simulink library "casper_library"  (Simulink 6.5)
PostLoadFcn:
  | % Stub definitions for mask variables
  | delay_depth=16;
  | n_bits=8;
  | bin_pt=7;
values from neighbouring files (symbols this model uses):
  add_latency = get_var('add_latency', 'defaults', defaults, varargin{:})    [butterfly_direct_init.m]    (also in fft_direct_init.m; fft_init.m; fft_wideband_real_init.m; pfb_real_add_tree_init.m)
  BitWidthIn = get_var('BitWidthIn', 'defaults', defaults, varargin{:})    [pfb_real_add_tree_init.m]
  blockCountBits = ceil(log2(numBlocks))    [address_gen_vacc_v2_mask.m]
  blockRowBits = 0    [address_gen_vacc_v2_mask.m]
  CoeffBitWidth = get_var('CoeffBitWidth', 'defaults', defaults, varargin{:})    [pfb_coeff_gen_init.m]    (also in pfb_real_add_tree_init.m)
  mult_latency = get_var('mult_latency', 'defaults', defaults, varargin{:})    [butterfly_direct_init.m]    (also in fft_direct_init.m; fft_init.m; fft_wideband_real_init.m)
  n_inputs = get_var('n_inputs', 'defaults', defaults, varargin{:})    [fft_init.m]    (also in fft_unscrambler_init.m; fft_wideband_real_init.m; partial_delay_init.m = get_var('n_inputs', varargin{:}); pfb_coeff_gen_init.m)
  PFBSize = get_var('PFBSize', 'defaults', defaults, varargin{:})    [pfb_coeff_gen_init.m]
undefined symbols (not defined in the file or in its folder): acc_len, ant_bits, bit_growth, cmult_4bit_br, cmult_4bit_em, cmult_4bit_sl, n_ants, n_bits_out, num_ants
libraries: xbsIndex_r3 x1646, xbsIndex_r4 x226, casper_library x156, xbsReplacements_r4 x17, xps_library x10, fft_library x4
(part 2 of 14)

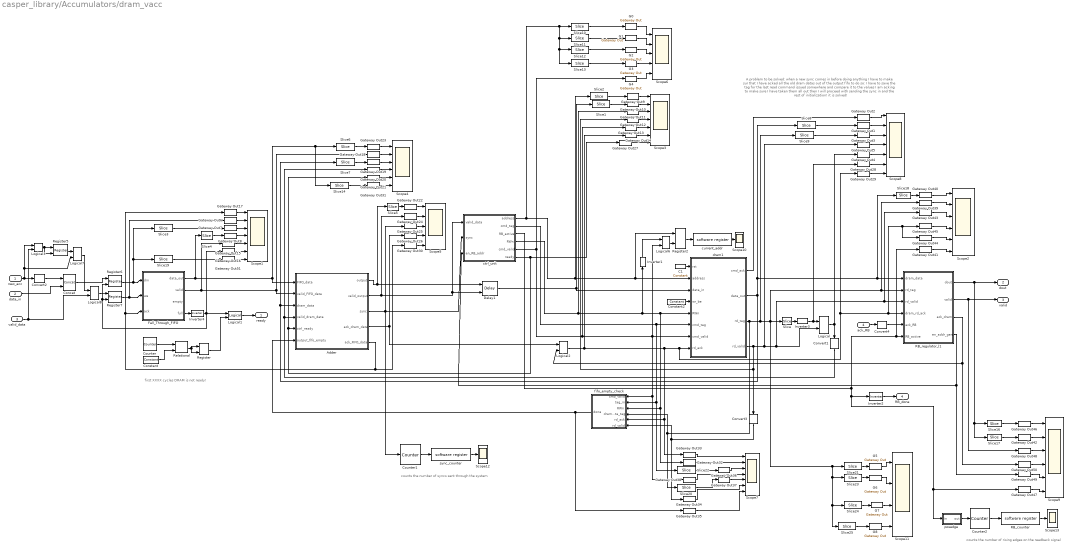
== system casper_library/Accumulators/dram_vacc ==
  note: A problem to be solved:
      | when a new sync comes in before doing anything I have to make sur
      | that I have acked all the old dram datas out of the output fifo
      | to do so: I have to save the tag for the last read command issued somewhere
      | and compare it to the values I am acking to make sure I have taken them all out
      | then I will proceed with sending the sync in and the rest of initialization!
      | it is solved!
  note: first XXXX cycles DRAM
      | is not ready!
  note: counts the number of syncs
      | sent through the system
  note: counts the number of rising edges on
      | the readback signal
  new_acc : Inport
  data_in : Inport  Port=2
  valid_data : Inport  Port=3
  ack_RB : Inport  Port=4
  Adder : Subsystem
  C1 : xbsIndex_r3/Constant  const=0  equ=P=C  arith_type=Boolean  n_bits=1  bin_pt=0  opselect=C  inp2=PCIN>>17  opr=+  inp1=P  carry=CIN  iostate=0  explicit_period=on  period=1  dbl_ovrd=off
  Concat : xbsIndex_r3/Concat  num_inputs=2  explicit_period=off  period=1  dbl_ovrd=off
  Constant : xbsIndex_r3/Constant  const=2^28-1  equ=P=C  arith_type=Unsigned  n_bits=28  bin_pt=0  opselect=C  inp2=PCIN>>17  opr=+  inp1=P  carry=CIN  iostate=0  explicit_period=on  period=1  dbl_ovrd=off
  Constant2 : xbsIndex_r3/Constant  const=2^18-1  equ=P=C  arith_type=Unsigned  n_bits=18  bin_pt=0  opselect=C  inp2=PCIN>>17  opr=+  inp1=P  carry=CIN  iostate=0  explicit_period=on  period=1  dbl_ovrd=off
  Convert1 : xbsIndex_r3/Convert  Orientation=down  arith_type=Boolean  n_bits=31  bin_pt=0  quantization=Truncate  overflow=Wrap  latency=0  explicit_period=off  period=1  dbl_ovrd=off  show_param=off  inserted_by_tool=off  pipeline=off
      settings: xl_area=[0, 0, 0, 0, 0, 0, 0]
  Convert2 : xbsIndex_r3/Convert  arith_type=Unsigned  n_bits=1  bin_pt=0  quantization=Truncate  overflow=Wrap  latency=0  explicit_period=off  period=1  dbl_ovrd=off  show_param=off  inserted_by_tool=off  pipeline=off
      settings: xl_area=[0, 0, 0, 0, 0, 0, 0]
  Convert3 : xbsIndex_r3/Convert  Orientation=down  arith_type=Boolean  n_bits=31  bin_pt=0  quantization=Truncate  overflow=Wrap  latency=0  explicit_period=off  period=1  dbl_ovrd=off  show_param=off  inserted_by_tool=off  pipeline=off
      settings: xl_area=[0, 0, 0, 0, 0, 0, 0]
  Convert4 : xbsIndex_r3/Convert  arith_type=Boolean  n_bits=31  bin_pt=0  quantization=Truncate  overflow=Wrap  latency=0  explicit_period=off  period=1  dbl_ovrd=off  show_param=off  inserted_by_tool=off  pipeline=off
      settings: xl_area=[0, 0, 0, 0, 0, 0, 0]
  Counter : xbsIndex_r3/Counter  cnt_type=Free Running  n_bits=28  bin_pt=0  arith_type=Unsigned  start_count=0  cnt_to=Inf  cnt_by_val=1  operation=Up  explicit_period=off  period=1  load_pin=off  rst=off  en=off  dbl_ovrd=off  show_param=off  use_rpm=on  gen_core=off
      settings: xl_area=[0, 0, 0, 0, 0, 0, 0]
  Counter1 : xbsIndex_r3/Counter  cnt_type=Free Running  n_bits=10  bin_pt=0  arith_type=Unsigned  start_count=0  cnt_to=Inf  cnt_by_val=1  operation=Up  explicit_period=off  period=1  load_pin=off  rst=off  en=on  dbl_ovrd=off  show_param=off  use_rpm=on  gen_core=off
      settings: xl_area=[0, 0, 0, 0, 0, 0, 0]
  Counter2 : xbsIndex_r3/Counter  cnt_type=Free Running  n_bits=10  bin_pt=0  arith_type=Unsigned  start_count=0  cnt_to=Inf  cnt_by_val=1  operation=Up  explicit_period=off  period=1  load_pin=off  rst=off  en=on  dbl_ovrd=off  show_param=off  use_rpm=on  gen_core=off
      settings: xl_area=[0, 0, 0, 0, 0, 0, 0]
  Delay1 : xbsIndex_r3/Delay  latency=1  reg_retiming=off  explicit_period=on  period=1  en=on  accept_only_valid=off  init_zero=on  dbl_ovrd=off  show_param=off
      settings: xl_area=[0, 0, 0, 0, 0, 0, 0]
  Fall_Through_FIFO : Subsystem
  G{0..8} (9 alike) : xbsIndex_r3/Gateway Out  output_type=Double  nbits=8  bin_pt=6  arith_type=Boolean  quantization=Truncate  overflow=Wrap  hdl_port=off  timing_constraint=None  locs_specified=off  LOCs={}  needs_fixed_name=off  show_param=off
      settings: xl_area=[0, 0, 0, 0, 0, 0, 0]
  Gateway Out{1..51} (51 alike) : xbsIndex_r3/Gateway Out  output_type=Double  nbits=8  bin_pt=6  arith_type=Boolean  quantization=Truncate  overflow=Wrap  hdl_port=off  timing_constraint=None  locs_specified=off  LOCs={}  needs_fixed_name=off  show_param=off
      settings: xl_area=[0, 0, 0, 0, 0, 0, 0]
  Inverter1 : xbsIndex_r3/Inverter  Orientation=up  latency=0  explicit_period=off  period=1  en=off  dbl_ovrd=off  show_param=off
      settings: xl_area=[0, 0, 0, 0, 0, 0, 0]
  Inverter2 : xbsIndex_r3/Inverter  latency=0  explicit_period=off  period=1  en=off  dbl_ovrd=off  show_param=off
      settings: xl_area=[0, 0, 0, 0, 0, 0, 0]
  Inverter3 : xbsIndex_r3/Inverter  latency=0  explicit_period=off  period=1  en=off  dbl_ovrd=off  show_param=off
      settings: xl_area=[0, 0, 0, 0, 0, 0, 0]
  Inverter4 : xbsIndex_r3/Inverter  latency=0  explicit_period=off  period=1  en=off  dbl_ovrd=off  show_param=off
      settings: xl_area=[0, 0, 0, 0, 0, 0, 0]
  Logical{,1,3,6,8} (5 alike) : xbsIndex_r3/Logical  logical_function=AND  inputs=2  precision=Full  arith_type=Unsigned  n_bits=8  bin_pt=2  align_bp=on  latency=0  explicit_period=off  period=1  en=off  dbl_ovrd=off  show_param=off
      settings: xl_area=[0, 0, 0, 0, 0, 0, 0]
  Logical2 : xbsIndex_r3/Logical  logical_function=OR  inputs=2  precision=Full  arith_type=Unsigned  n_bits=8  bin_pt=2  align_bp=on  latency=0  explicit_period=off  period=1  en=off  dbl_ovrd=off  show_param=off
      settings: xl_area=[0, 0, 0, 0, 0, 0, 0]
  Logical7 : xbsIndex_r3/Logical  logical_function=OR  inputs=2  precision=Full  arith_type=Unsigned  n_bits=8  bin_pt=2  align_bp=on  latency=0  explicit_period=off  period=1  en=off  dbl_ovrd=off  show_param=off
      settings: xl_area=[0, 0, 0, 0, 0, 0, 0]
  RB_counter : xps_library/software register  Tag=xps:sw_reg  io_dir=To Processor  arith_type=Unsigned  bitwidth=32  bin_pt=0  sample_period=1  gw_name=casper_library_Accumulators_dram_vacc_RB_counter_user_data_in
  RB_regulator_l1 : Subsystem
  Register{,2,5..7} (5 alike) : xbsIndex_r3/Register  init=0  reg_only_valid=off  explicit_period=off  period=1  rst=off  en=on  out_en=off  dbl_ovrd=off  show_param=off
      settings: xl_area=[0, 0, 0, 0, 0, 0, 0]
  Relational : xbsIndex_r3/Relational  mode=a=b  latency=1  explicit_period=off  period=1  en=off  dbl_ovrd=off  show_param=off
      settings: xl_area=[0, 0, 0, 0, 0, 0, 0]
  Scope{1,3,7..8} (4 alike) : Scope  NumInputPorts=7
      Scope1 settings: TimeRange=400000  YMin=0~0~0~0~0~0~0  YMax=1~1~400~400~1~2~1  SaveName=ScopeData7
      Scope3 settings: YMin=0~0~0~0~0~0~0  YMax=150~2500~1~1~1~1~1  SaveName=ScopeData6
      Scope7 settings: YMin=0~0~0~0~0~0.95~0  YMax=1~1100~7500~1~1~1.05~1  SaveName=ScopeData17
      Scope8 settings: YMin=0~0~2.68438e+008~0~0~0~0  YMax=1~11000~2.68439e+008~1~1~1~1  SaveName=ScopeData19
  Scope10 : Scope
      settings: YMin=0  YMax=100  SaveName=ScopeData27
  Scope11 : Scope  NumInputPorts=4
      settings: YMin=0~0~0~0  YMax=200~4000~1~1  SaveName=ScopeData28
  Scope12 : Scope
      settings: YMin=0  YMax=100  SaveName=ScopeData32
  Scope13 : Scope
      settings: YMin=0  YMax=100  SaveName=ScopeData33
  Scope2 : Scope  NumInputPorts=6
      settings: YMin=-1~0.95~-1~-1~0.95~-1  YMax=1~1.05~1~1~1.05~1  SaveName=ScopeData22
  Scope4 : Scope  NumInputPorts=6
      settings: YMin=0.95~0.95~-1~-1~0.95~-1  YMax=1.05~1.05~1~1~1.05~1  SaveName=ScopeData8
  Scope5 : Scope  NumInputPorts=5
      settings: YMin=0~0~-1~0~0  YMax=250~1~1~1~1  SaveName=ScopeData9
  Scope6 : Scope  NumInputPorts=5
      settings: YMin=0~0~0~0~0  YMax=200~4000~1~1~1  SaveName=ScopeData14
  Scope9 : Scope  NumInputPorts=6
      settings: YMin=1.9~1.9~-1~0~-1~0.95  YMax=2.1~2.1~1~1~1~1.05  SaveName=ScopeData23
  Slice : xbsIndex_r3/Slice  mode=Upper Bit Location + Width  nbits=1  bit1=0  base1=MSB of Input  bit0=0  base0=LSB of Input  boolean_output=off  explicit_period=off  period=1  dbl_ovrd=off
  Slice{1,3..8,16..18} (10 alike) : xbsIndex_r3/Slice  mode=Lower Bit Location + Width  nbits=32  bit1=0  base1=MSB of Input  bit0=0  base0=LSB of Input  boolean_output=off  explicit_period=off  period=1  dbl_ovrd=off
  Slice{2,10,20..22} (5 alike) : xbsIndex_r3/Slice  mode=Lower Bit Location + Width  nbits=8  bit1=0  base1=MSB of Input  bit0=5  base0=LSB of Input  boolean_output=off  explicit_period=off  period=1  dbl_ovrd=off
  Slice11 : xbsIndex_r3/Slice  mode=Lower Bit Location + Width  nbits=14  bit1=0  base1=MSB of Input  bit0=14  base0=LSB of Input  boolean_output=off  explicit_period=off  period=1  dbl_ovrd=off
  Slice12 : xbsIndex_r3/Slice  mode=Lower Bit Location + Width  nbits=1  bit1=0  base1=MSB of Input  bit0=13  base0=LSB of Input  boolean_output=off  explicit_period=off  period=1  dbl_ovrd=off
  Slice13 : xbsIndex_r3/Slice  mode=Lower Bit Location + Width  nbits=2  bit1=0  base1=MSB of Input  bit0=28  base0=LSB of Input  boolean_output=off  explicit_period=off  period=1  dbl_ovrd=off
  Slice14 : xbsIndex_r3/Slice  mode=Upper Bit Location + Width  nbits=1  bit1=0  base1=MSB of Input  bit0=0  base0=LSB of Input  boolean_output=off  explicit_period=off  period=1  dbl_ovrd=off
  Slice19 : xbsIndex_r3/Slice  mode=Upper Bit Location + Width  nbits=1  bit1=0  base1=MSB of Input  bit0=0  base0=LSB of Input  boolean_output=off  explicit_period=off  period=1  dbl_ovrd=off
  Slice23 : xbsIndex_r3/Slice  mode=Lower Bit Location + Width  nbits=14  bit1=0  base1=MSB of Input  bit0=14  base0=LSB of Input  boolean_output=off  explicit_period=off  period=1  dbl_ovrd=off
  Slice24 : xbsIndex_r3/Slice  mode=Lower Bit Location + Width  nbits=1  bit1=0  base1=MSB of Input  bit0=13  base0=LSB of Input  boolean_output=off  explicit_period=off  period=1  dbl_ovrd=off
  Slice25 : xbsIndex_r3/Slice  mode=Lower Bit Location + Width  nbits=2  bit1=0  base1=MSB of Input  bit0=28  base0=LSB of Input  boolean_output=off  explicit_period=off  period=1  dbl_ovrd=off
  Slice9 : xbsIndex_r3/Slice  mode=Lower Bit Location + Width  nbits=31  bit1=0  base1=MSB of Input  bit0=0  base0=LSB of Input  boolean_output=off  explicit_period=off  period=1  dbl_ovrd=off
  ctrl_unit : Subsystem  mask{burst_length=valid_length, acc_length=acc_length}
      mask prompts: burst_length "Burst Length?"; acc_length "Accumulation length?"
  current_addr : xps_library/software register  Tag=xps:sw_reg  io_dir=To Processor  arith_type=Unsigned  bitwidth=32  bin_pt=0  sample_period=1  gw_name=casper_library_Accumulators_dram_vacc_current_addr_user_data_in
  dram1 : Subsystem  Tag=xps:dram  AncestorBlock=xps_library/dram  mask(dram){dimm=1, arith_type=Unsigned, bin_pt=0, ip_clock=200, sample_period=1, use_sim=on, bank_mgt=on, wide_data=off, half_burst=off, shared=on}
      mask prompts: arith_type "Data Type"; bin_pt "Data binary point"; ip_clock "Datapath clock rate (MHz)"; sample_period "Sample period"; use_sim "Simulate DRAM using ModelSim"; bank_mgt "Enable bank management"; wide_data "Use wide data bus (288 bits)"; half_burst "Use half-burst"; shared "Share with PowerPC"
      mask help:
      | Interface to 1GB DDR2 DIMMs on BEE2.
      |
      | To simulate using ModelSim, place a ModelSim block named 'ModelSim' (case-sensitive) in the top level of the design.
      mask init:
      | dram_mask;
      mask StyleString: popup(1|2|3|4),popup(Boolean|Unsigned|Signed  (2's comp)),edit,edit,edit,checkbox,checkbox,checkbox,checkbox,checkbox
      mask CallbackString:
      | |||||||myname=gcb;
      | if strcmp(get_param(myname, 'wide_data'), 'off')
      |     set_param(myname, 'MaskEnables', {'on','on','on','on','on','on','on','on','on','on'});
      | else
      |     set_param(myname, 'half_burst', 'off');
      |     set_param(myname, 'MaskEnables', {'on','on','on','on','on','on','on','on','off','on'});
      | end||
  fifo_empty_check : Subsystem  Orientation=left
  posedge : Subsystem
  sync_counter : xps_library/software register  Tag=xps:sw_reg  io_dir=To Processor  arith_type=Unsigned  bitwidth=32  bin_pt=0  sample_period=1  gw_name=casper_library_Accumulators_dram_vacc_sync_counter_user_data_in
  ready : Outport
  dout : Outport  Port=2
  valid : Outport  Port=3
  RB_done : Outport  Port=4
  wires:
  Logical8/1 -> Register7/1
  Concat/1 -> Register6/1
  Logical3/1 -> Register5/2, Register5/1
  Logical7/1 -> Logical8/1
  Register5/1 -> Logical7/1
  Convert2/1 -> Concat/1
  valid_data/1 -> Logical8/2, Logical3/2
  data_in/1 -> Concat/2
  new_acc/1 -> Logical3/1, Logical7/2, Convert2/1
  Adder/4(ack_dram_data) -> Gateway Out26/1, Logical2/1
  Fall_Through_FIFO/1(data_out) -> Adder/1(FIFO_data), Slice6/1, Slice14/1, Slice4/1
  Fall_Through_FIFO/2(valid) -> Gateway Out15/1, Gateway Out18/1, Adder/2(valid_FIFO_data)
  ctrl_unit/1(address) -> Slice10/1, Slice11/1, Slice13/1, Slice12/1, Slice2/1, dram1/2(address), Register2/1
  ctrl_unit/4(RWn) -> Gateway Out11/1, dram1/5(RWn), fifo_empty_check/3(RWn), Gateway Out32/1, Inverter1/1
  C1/1 -> dram1/1(rst)
  Constant2/1 -> dram1/4(wr_be)
  Adder/1(output) -> Slice5/1, Delay1/1
  dram1/2(data_out) -> Slice7/1, Adder/3(dram_data), Slice8/1, Slice18/1, RB_regulator_l1/1(dram_data)
  dram1/3(rd_tag) -> Slice9/1, Slice/1, Slice21/1, Slice23/1, Slice25/1, Slice24/1, Gateway Out39/1, RB_regulator_l1/2(rd_tag), fifo_empty_check/4(dram_data_tag), Slice20/1
  Slice/1 -> Inverter3/1
  dram1/4(rd_valid) -> Gateway Out5/1, Logical/2, Gateway Out43/1, RB_regulator_l1/3(rd_valid), Gateway Out12/1, Convert3/1
  Logical/1 -> Gateway Out4/1, Convert1/1
  ctrl_unit/6(ready) -> Gateway Out21/1, Adder/5(ctrl_ready), Gateway Out27/1
  Adder/2(valid_output) -> ctrl_unit/1(valid_data), Delay1/2, Gateway Out24/1
  Adder/3(sync) -> Gateway Out25/1, Counter1/1, ctrl_unit/2(sync)
  dram1/1(cmd_ack) -> Gateway Out2/1
  ctrl_unit/2(cmd_tag) -> dram1/6(cmd_tag), fifo_empty_check/2(tag_in), Slice22/1
  Fall_Through_FIFO/4(full) -> Inverter4/1
  Register6/1 -> Fall_Through_FIFO/1(din), Slice3/1, Slice19/1
  Gateway Out9/1 -> Scope3/1
  Gateway Out10/1 -> Scope3/2
  Gateway Out11/1 -> Scope3/3
  Gateway Out12/1 -> Scope3/4
  Gateway Out13/1 -> Scope3/5
  Gateway Out14/1 -> Scope3/6
  Slice1/1 -> Gateway Out10/1
  Slice2/1 -> Gateway Out9/1
  Gateway Out17/1 -> Scope1/1
  Gateway Out6/1 -> Scope1/2
  Gateway Out7/1 -> Scope1/3
  Gateway Out8/1 -> Scope1/4
  Gateway Out15/1 -> Scope1/5
  Gateway Out16/1 -> Scope1/6
  Gateway Out23/1 -> Scope4/1
  Gateway Out18/1 -> Scope4/2
  Gateway Out19/1 -> Scope4/3
  Gateway Out20/1 -> Scope4/4
  Gateway Out21/1 -> Scope4/5
  Gateway Out22/1 -> Scope5/1
  Gateway Out24/1 -> Scope5/2
  Gateway Out25/1 -> Scope5/3
  Gateway Out26/1 -> Scope5/4
  Slice3/1 -> Gateway Out7/1
  Slice4/1 -> Gateway Out8/1
  Convert1/1 -> Gateway Out20/1, Adder/4(valid_dram_data)
  Slice5/1 -> Gateway Out22/1
  Slice6/1 -> Gateway Out23/1
  Slice7/1 -> Gateway Out19/1
  Gateway Out27/1 -> Scope3/7
  Slice8/1 -> Gateway Out1/1
  Slice9/1 -> Gateway Out3/1
  Adder/5(ack_FIFO_data) -> Fall_Through_FIFO/3(ack), Gateway Out17/1, Gateway Out30/1
  Gateway Out30/1 -> Scope5/5
  Slice10/1 -> G0/1
  Slice11/1 -> G1/1
  Slice12/1 -> G2/1
  Slice13/1 -> G3/1
  G0/1 -> Scope6/1
  G1/1 -> Scope6/2
  G2/1 -> Scope6/3
  G3/1 -> Scope6/4
  G4/1 -> Scope6/5
  Gateway Out31/1 -> Scope4/6
  Slice14/1 -> Gateway Out31/1
  Delay1/1 -> dram1/3(data_in), Slice1/1
  fifo_empty_check/1(done) -> Adder/6(output_fifo_empty), Gateway Out35/1
  Gateway Out33/1 -> Scope7/1
  Gateway Out32/1 -> Scope7/2
  Gateway Out36/1 -> Scope7/3
  Gateway Out37/1 -> Scope7/5
  Gateway Out38/1 -> Scope7/4
  Gateway Out34/1 -> Scope7/6
  Gateway Out35/1 -> Scope7/7
  Gateway Out2/1 -> Scope8/1
  Gateway Out1/1 -> Scope8/2
  Gateway Out3/1 -> Scope8/3
  Gateway Out5/1 -> Scope8/4
  Gateway Out4/1 -> Scope8/5
  Gateway Out28/1 -> Scope8/6
  Gateway Out29/1 -> Scope8/7
  RB_regulator_l1/1(dout) -> dout/1, Slice16/1, Slice17/1
  RB_regulator_l1/2(valid) -> Gateway Out48/1, valid/1
  RB_regulator_l1/3(ack_dram) -> Gateway Out50/1, Logical2/2
  RB_regulator_l1/4(en_addr_gen) -> ctrl_unit/3(en_RB_addr), Gateway Out49/1
  ctrl_unit/3(RB_active) -> Gateway Out41/1, RB_regulator_l1/6(RB_active), Gateway Out47/1, posedge/1(in), Inverter2/1
  Logical2/1 -> fifo_empty_check/5(rd_ack), Gateway Out33/1, dram1/8(rd_ack), Gateway Out29/1, RB_regulator_l1/4(dram_rd_ack), Gateway Out45/1, Gateway Out44/1, Gateway Out14/1
  Gateway Out40/1 -> Scope2/1
  Gateway Out39/1 -> Scope2/2
  Gateway Out43/1 -> Scope2/3
  Gateway Out45/1 -> Scope2/4
  Gateway Out44/1 -> Scope2/5
  Gateway Out41/1 -> Scope2/6
  Gateway Out46/1 -> Scope9/1
  Gateway Out42/1 -> Scope9/2
  Gateway Out48/1 -> Scope9/3
  Gateway Out50/1 -> Scope9/4
  Gateway Out49/1 -> Scope9/5
  Convert3/1 -> fifo_empty_check/6(rd_valid), Gateway Out34/1
  Slice16/1 -> Gateway Out46/1
  Slice17/1 -> Gateway Out42/1
  Slice18/1 -> Gateway Out40/1
  Gateway Out47/1 -> Scope9/6
  Logical1/1 -> ready/1
  Counter/1 -> Relational/1
  Constant/1 -> Relational/2
  Relational/1 -> Register/1, Register/2
  Register/1 -> Logical1/2
  Register7/1 -> Fall_Through_FIFO/2(we), Gateway Out6/1
  Gateway Out51/1 -> Scope1/7
  Slice19/1 -> Gateway Out51/1
  Register2/1 -> current_addr/1
  Logical6/1 -> Register2/2
  Inverter1/1 -> Logical6/1
  current_addr/1 -> Scope10/1
  Slice22/1 -> Gateway Out36/1
  Slice20/1 -> Gateway Out37/1
  Slice21/1 -> G5/1
  Slice23/1 -> G6/1
  Slice24/1 -> G7/1
  Slice25/1 -> G8/1
  G5/1 -> Scope11/1
  G6/1 -> Scope11/2
  G7/1 -> Scope11/3
  G8/1 -> Scope11/4
  Inverter4/1 -> Register6/2, Register7/2, Gateway Out16/1, Logical1/1
  Counter1/1 -> sync_counter/1
  sync_counter/1 -> Scope12/1
  Counter2/1 -> RB_counter/1
  RB_counter/1 -> Scope13/1
  posedge/1(out) -> Counter2/1
  Inverter2/1 -> RB_done/1
  ctrl_unit/5(cmd_valid) -> Gateway Out13/1, dram1/7(cmd_valid), fifo_empty_check/1(cmd_valid), Gateway Out38/1, Logical6/2, G4/1
  ack_RB/1 -> Convert4/1
  Inverter3/1 -> Logical/1, Gateway Out28/1
  Convert4/1 -> RB_regulator_l1/5(ack_RB)

== system casper_library/Correlator/baseline_tap ==
  a_del : Inport
  a_ndel : Inport  Port=2
  a_end : Inport  Port=3
  acc_in : Inport  Port=4
  valid_in : Inport  Port=5
  rst : Inport  Port=6
  sync1 : Inport  Port=7
  Constant : xbsIndex_r3/Constant  const=ant_sep * acc_len  equ=P=C  arith_type=Unsigned  n_bits=ant_bits + bit_growth  bin_pt=0  opselect=C  inp2=PCIN>>17  opr=+  inp1=P  carry=CIN  iostate=0  explicit_period=off  period=1  dbl_ovrd=off
  Convert : xbsIndex_r3/Convert  arith_type=Unsigned  n_bits=1  bin_pt=0  quantization=Truncate  overflow=Wrap  latency=0  explicit_period=off  period=1  dbl_ovrd=off  show_param=off  inserted_by_tool=off  pipeline=off
      settings: xl_area=[0, 0, 0, 0, 0, 0, 0]
  Counter : xbsIndex_r3/Counter  cnt_type=Count Limited  n_bits=ant_bits + bit_growth  bin_pt=0  arith_type=Unsigned  start_count=0  cnt_to=n_ants * acc_len - 1  cnt_by_val=1  operation=Up  explicit_period=off  period=1  load_pin=off  rst=on  en=off  dbl_ovrd=off  show_param=off  use_rpm=on  gen_core=off
      settings: xl_area=[0, 0, 0, 0, 0, 0, 0]
  Delay1 : xbsIndex_r3/Delay  latency=1  reg_retiming=off  explicit_period=off  period=1  en=off  accept_only_valid=off  init_zero=on  dbl_ovrd=off  show_param=off
      settings: xl_area=[0, 0, 0, 0, 0, 0, 0]
  Delay3 : xbsIndex_r3/Delay  latency=1  reg_retiming=off  explicit_period=off  period=1  en=off  accept_only_valid=off  init_zero=on  dbl_ovrd=off  show_param=off
      settings: xl_area=[0, 0, 0, 0, 0, 0, 0]
  Delay7 : xbsIndex_r3/Delay  latency=1  reg_retiming=off  explicit_period=on  period=1  en=off  accept_only_valid=off  init_zero=on  dbl_ovrd=off  show_param=off
      settings: xl_area=[0, 0, 0, 0, 0, 0, 0]
  Delay8 : xbsIndex_r3/Delay  latency=1  reg_retiming=off  explicit_period=on  period=1  en=off  accept_only_valid=off  init_zero=on  dbl_ovrd=off  show_param=off
      settings: xl_area=[0, 0, 0, 0, 0, 0, 0]
  Mux : xbsIndex_r3/Mux  inputs=2  precision=Full  arith_type="Signed  (2's comp)"  n_bits=8  bin_pt=2  quantization=Truncate  overflow=Wrap  latency=1  explicit_period=off  period=1  en=off  dbl_ovrd=off  show_param=off  mux_type=off  use_rpm=off  gen_core=off
      settings: xl_area=[0, 0, 0, 0, 0, 0, 0]
  Relational : xbsIndex_r3/Relational  mode=a<b  latency=0  explicit_period=off  period=1  en=off  dbl_ovrd=off  show_param=off
      settings: xl_area=[0, 0, 0, 0, 0, 0, 0]
  delay : Subsystem  BlockChoice=delay_bram
      link override delay_bram: DelayLen=acc_len  bram_latency=bram_latency
      link override delay_slr: DelayLen=acc_len
      settings: AttributesFormatString=%<BlockChoice>  TemplateBlock=casper_library/Delays/delay  MemberBlocks=delay_bram,delay_slr
  dual_pol_cmac : Subsystem
  a_del_out : Outport
  a_ndel_out : Outport  Port=2
  a_end_out : Outport  Port=3
  acc_out : Outport  Port=4
  valid_out : Outport  Port=5
  rst_out : Outport  Port=6
  sync_out : Outport  Port=7
  wires:
  sync1/1 -> sync_out/1
  Delay1/1 -> rst_out/1, dual_pol_cmac/4(sync)
  Delay8/1 -> a_end_out/1
  Delay7/1 -> a_ndel_out/1
  Delay3/1 -> a_del_out/1, dual_pol_cmac/1(a1)
  a_end/1 -> Delay8/1, Mux/3
  a_ndel/1 -> Delay7/1, Mux/2
  valid_in/1 -> dual_pol_cmac/5(valid_in)
  dual_pol_cmac/2(valid_out) -> valid_out/1
  acc_in/1 -> dual_pol_cmac/3(acc_in)
  dual_pol_cmac/1(acc_out) -> acc_out/1
  a_del/1 -> delay/1(In1)
  rst/1 -> Counter/1, Delay1/1
  Convert/1 -> Mux/1
  Relational/1 -> Convert/1
  Constant/1 -> Relational/2
  Counter/1 -> Relational/1
  Mux/1 -> dual_pol_cmac/2(a2)
  delay/1(Out1) -> Delay3/1

== system casper_library/Correlator/x_engine ==
  ant : Inport
  sync_in : Inport  Port=2
  Constant : xbsIndex_r3/Constant  const=0  equ=P=C  arith_type=Unsigned  n_bits=8 * n_bits_out  bin_pt=0  opselect=C  inp2=PCIN>>17  opr=+  inp1=P  carry=CIN  iostate=0  explicit_period=on  period=1  dbl_ovrd=off
  Constant1 : xbsIndex_r3/Constant  const=0  equ=P=C  arith_type=Boolean  n_bits=1  bin_pt=0  opselect=C  inp2=PCIN>>17  opr=+  inp1=P  carry=CIN  iostate=0  explicit_period=on  period=1  dbl_ovrd=off
  Term1 : Terminator
  Term2 : Terminator
  Term3 : Terminator
  auto_tap : Subsystem  mask(auto_tap){use_ded_mult=1}
      mask prompts: use_ded_mult "Use Dedicated Multipliers"
      mask init:
      | auto_tap_init(gcb, ...
      |     'use_ded_mult', use_ded_mult);
      settings: AttributesFormatString=mult=1
  baseline_tap1 : casper_library/Correlator/baseline_tap  ant_sep=1  use_ded_mult=1  use_bram_delay=1
      settings: AttributesFormatString=ant_sep=1, mult=1, bram=1
  baseline_tap2 : casper_library/Correlator/baseline_tap  ant_sep=2  use_ded_mult=1  use_bram_delay=1
      settings: AttributesFormatString=ant_sep=2, mult=1, bram=1
  acc : Outport
  valid : Outport  Port=2
  sync_out : Outport  Port=3
  wires:
  ant/1 -> auto_tap/1(a_del), auto_tap/2(a_ndel)
  Constant/1 -> auto_tap/4(acc_in)
  Constant1/1 -> auto_tap/5(valid_in)
  sync_in/1 -> auto_tap/6(sync_in)
  auto_tap/1(a_del_out) -> baseline_tap1/1
  auto_tap/2(a_ndel_out) -> baseline_tap1/2
  auto_tap/3(a_end_out) -> baseline_tap1/3
  auto_tap/4(acc_out) -> baseline_tap1/4
  auto_tap/5(valid_out) -> baseline_tap1/5
  auto_tap/6(rst_out) -> baseline_tap1/6
  auto_tap/7(sync_out) -> baseline_tap1/7
  baseline_tap1/1 -> baseline_tap2/1
  baseline_tap1/2 -> baseline_tap2/2
  baseline_tap1/3 -> baseline_tap2/3
  baseline_tap1/4 -> baseline_tap2/4
  baseline_tap1/5 -> baseline_tap2/5
  baseline_tap1/6 -> baseline_tap2/6
  baseline_tap1/7 -> baseline_tap2/7
  baseline_tap2/1 -> auto_tap/3(a_loop)
  baseline_tap2/2 -> Term1/1
  baseline_tap2/3 -> Term2/1
  baseline_tap2/4 -> acc/1
  baseline_tap2/5 -> valid/1
  baseline_tap2/6 -> Term3/1
  baseline_tap2/7 -> sync_out/1

== system casper_library/Correlator/x_engine_reorder ==
  acc : Inport
  valid : Inport  Port=2
  window_valid : Inport  Port=3
  sync : Inport  Port=4
  Constant4 : xbsIndex_r3/Constant  const=0  equ=P=C  arith_type=Boolean  n_bits=elements_bits + 1  bin_pt=0  opselect=C  inp2=PCIN>>17  opr=+  inp1=P  carry=CIN  iostate=0  explicit_period=on  period=1  dbl_ovrd=off
  Counter1 : xbsIndex_r3/Counter  cnt_type=Count Limited  n_bits=elements_bits + 1  bin_pt=0  arith_type=Unsigned  start_count=0  cnt_to=2 * num_elements - 1  cnt_by_val=1  operation=Up  explicit_period=off  period=1  load_pin=off  rst=on  en=on  dbl_ovrd=off  show_param=off  use_rpm=on  gen_core=off
      settings: xl_area=[0, 0, 0, 0, 0, 0, 0]
  Delay{1..3,6,8} (5 alike) : xbsIndex_r3/Delay  latency=1  reg_retiming=off  explicit_period=off  period=1  en=off  accept_only_valid=off  init_zero=on  dbl_ovrd=off  show_param=off
      settings: xl_area=[0, 0, 0, 0, 0, 0, 0]
  Dual Port RAM : xbsIndex_r3/Dual Port RAM  depth=num_elements * 2  initVector=0  write_mode_A=Read After Write  write_mode_B=No Read On Write  latency=1  mem_collision=off  init_zero=on  explicit_period=off  period=1  dbl_ovrd=off  rst_a=off  init_a=0  rst_b=off  init_b=0  show_param=off  distributed_mem=off  use_rpm=off  gen_core=off
      settings: xl_area=[0, 0, 0, 0, 0, 0, 0]
  Logical{,1,4,7} (4 alike) : xbsIndex_r3/Logical  logical_function=OR  inputs=2  precision=Full  arith_type=Unsigned  n_bits=8  bin_pt=2  align_bp=on  latency=0  explicit_period=off  period=1  en=off  dbl_ovrd=off  show_param=off
      settings: xl_area=[0, 0, 0, 0, 0, 0, 0]
  Mux : xbsIndex_r3/Mux  inputs=2  precision=Full  arith_type="Signed  (2's comp)"  n_bits=8  bin_pt=2  quantization=Truncate  overflow=Wrap  latency=0  explicit_period=off  period=1  en=off  dbl_ovrd=off  show_param=off  mux_type=off  use_rpm=off  gen_core=off
      settings: xl_area=[0, 0, 0, 0, 0, 0, 0]
  Terminator : Terminator
  posedge : casper_library/Misc/posedge  Tag=Rising Edge Detector
  sync_delay_en : casper_library/Delays/sync_delay_en  DelayLen=num_elements
  win1_ctrl : Subsystem
  win2_ctrl : Subsystem
  x_engine_valid_mask : Subsystem  mask{num_ants=num_ants}
      mask prompts: num_ants "Number of Antennas"
      mask init:
      | num_taps = floor(num_ants/2) + 1;
      | cntr_bits = floor(log2(num_taps)) + 1;
      | ant_bits = floor(log2(num_ants)) + 1;
      | num_validins = num_ants*num_taps;
      | validin_bits = floor(log2(num_validins)) + 1;
  acc_out : Outport
  valid_out : Outport  Port=2
  sync_out : Outport  Port=3
  wires:
  Delay3/1 -> Logical4/1, sync_delay_en/1, win1_ctrl/3(sync), win2_ctrl/3(sync)
  x_engine_valid_mask/2(write_w2) -> win2_ctrl/1(write), Logical1/1, Mux/1
  x_engine_valid_mask/1(write_win1) -> Logical1/2, win1_ctrl/1(write), Logical4/2
  valid/1 -> x_engine_valid_mask/1(valid_in)
  sync/1 -> Delay3/1, x_engine_valid_mask/2(sync)
  Logical/1 -> Counter1/2
  Mux/1 -> Dual Port RAM/1
  Counter1/1 -> Dual Port RAM/4
  Delay8/1 -> Dual Port RAM/2, Dual Port RAM/5
  acc/1 -> Delay8/1
  Dual Port RAM/1 -> Terminator/1
  Dual Port RAM/2 -> acc_out/1
  Constant4/1 -> Dual Port RAM/6
  Delay1/1 -> valid_out/1
  Delay2/1 -> sync_out/1
  Logical1/1 -> Dual Port RAM/3
  Logical4/1 -> sync_delay_en/2
  sync_delay_en/1 -> posedge/1
  posedge/1 -> Delay2/1, Counter1/1
  window_valid/1 -> Delay6/1
  win1_ctrl/3(read_valid) -> Logical7/1
  win2_ctrl/3(read_valid) -> Logical7/2
  Logical7/1 -> Delay1/1
  win2_ctrl/1(write_addr) -> Mux/3
  win2_ctrl/2(read) -> Logical/2
  win1_ctrl/1(write_addr) -> Mux/2
  win1_ctrl/2(read) -> Logical/1
  Delay6/1 -> win1_ctrl/2(win_valid), win2_ctrl/2(win_valid)

== system casper_library/Delays/delay ==
  In1 : Inport
  delay_bram : casper_library/Delays/delay_bram  SystemSampleTime=-1  DelayLen=7  bram_latency=4
  Out1 : Outport
  wires:
  In1/1 -> delay_bram/1
  delay_bram/1 -> Out1/1

== system casper_library/Delays/delay_bram ==
  In1 : Inport
  Constant2 : xbsIndex_r4/Constant  arith_type=Boolean  const=1  n_bits=1  bin_pt=0  explicit_period=on  period=1  equ=P=C  opselect=C  inp2=PCIN>>17  opr=+  inp1=P  carry=CIN  dbl_ovrd=off  block_type=constant
      settings: block_version=9.1.01
  Counter : xbsIndex_r4/Counter  cnt_type=Count Limited  cnt_to=DelayLen - bram_latency - 1  operation=Up  start_count=0  cnt_by_val=1  arith_type=Unsigned  n_bits=BitWidth  bin_pt=0  load_pin=off  rst=off  en=off  explicit_period=off  period=1  dbl_ovrd=off  use_behavioral_HDL=off  use_rpm=off  block_type=counter
      settings: xl_area=[0, 0, 0, 0, 0, 0, 0]  block_version=9.1.01
  Single Port RAM : xbsIndex_r4/Single Port RAM  depth=2^BitWidth  initVector=0  distributed_mem=Block RAM  write_mode=Read Before Write  rst=off  init_reg=0  en=off  latency=bram_latency  dbl_ovrd=off  optimize=Area  use_rpm=off  block_type=spram
      settings: xl_area=[0, 0, 0, 0, 0, 0, 0]  block_version=9.1.01
  Out1 : Outport
  wires:
  Constant2/1 -> Single Port RAM/3
  In1/1 -> Single Port RAM/2
  Counter/1 -> Single Port RAM/1
  Single Port RAM/1 -> Out1/1

== system casper_library/Delays/delay_bram_en_plus ==
  din : Inport
  en : Inport  Port=2
  Counter : xbsIndex_r4/Counter  cnt_type=Count Limited  cnt_to=DelayLen - 1  operation=Up  start_count=0  cnt_by_val=1  arith_type=Unsigned  n_bits=BitWidth  bin_pt=0  load_pin=off  rst=off  en=on  explicit_period=off  period=1  dbl_ovrd=off  use_behavioral_HDL=off  use_rpm=off  block_type=counter
      settings: xl_area=[0, 0, 0, 0, 0, 0, 0]  block_version=9.1.01
  Delay : xbsIndex_r4/Delay  en=off  latency=bram_latency  dbl_ovrd=off  reg_retiming=off  block_type=delay
      settings: xl_area=[0, 0, 0, 0, 0, 0, 0]  block_version=9.1.01
  Single Port RAM : xbsIndex_r4/Single Port RAM  depth=2^BitWidth  initVector=0  distributed_mem=Block RAM  write_mode=Read Before Write  rst=off  init_reg=0  en=off  latency=bram_latency  dbl_ovrd=off  optimize=Area  use_rpm=off  block_type=spram
      settings: xl_area=[0, 0, 0, 0, 0, 0, 0]  block_version=9.1.01
  dout : Outport
  valid : Outport  Port=2
  wires:
  Delay/1 -> valid/1
  en/1 -> Delay/1, Counter/1, Single Port RAM/3
  din/1 -> Single Port RAM/2
  Counter/1 -> Single Port RAM/1
  Single Port RAM/1 -> dout/1

== system casper_library/Delays/delay_bram_prog ==
  din : Inport
  delay : Inport  Port=2
  AddSub : xbsIndex_r4/AddSub  mode=Subtraction  use_carryin=off  use_carryout=off  en=off  latency=2  precision=User Defined  arith_type=Unsigned  n_bits=MaxDelay  bin_pt=0  quantization=Truncate  overflow=Wrap  dbl_ovrd=off  use_behavioral_HDL=on  pipelined=off  use_rpm=on  block_type=addsub
      settings: xl_area=[0, 0, 0, 0, 0, 0, 0]  block_version=9.1.01
  Constant1 : xbsIndex_r4/Constant  arith_type=Unsigned  const=bram_latency + 1  n_bits=MaxDelay  bin_pt=0  explicit_period=on  period=1  equ=P=C  opselect=C  inp2=PCIN>>17  opr=+  inp1=P  carry=CIN  dbl_ovrd=off  block_type=constant
      settings: block_version=9.1.01
  Constant2 : xbsIndex_r4/Constant  arith_type=Boolean  const=1  n_bits=1  bin_pt=0  explicit_period=on  period=1  equ=P=C  opselect=C  inp2=PCIN>>17  opr=+  inp1=P  carry=CIN  dbl_ovrd=off  block_type=constant
      settings: block_version=9.1.01
  Counter : xbsIndex_r4/Counter  cnt_type=Free Running  cnt_to=inf  operation=Up  start_count=0  cnt_by_val=1  arith_type=Unsigned  n_bits=MaxDelay  bin_pt=0  load_pin=off  rst=on  en=off  explicit_period=on  period=1  dbl_ovrd=off  use_behavioral_HDL=off  use_rpm=off  block_type=counter
      settings: xl_area=[0, 0, 0, 0, 0, 0, 0]  block_version=9.1.01
  Relational : xbsIndex_r4/Relational  mode=a>=b  en=off  latency=0  dbl_ovrd=off  block_type=relational
      settings: xl_area=[0, 0, 0, 0, 0, 0, 0]  block_version=9.1.01
  Single Port RAM : xbsIndex_r4/Single Port RAM  depth=2^MaxDelay  initVector=0  distributed_mem=Block RAM  write_mode=Read Before Write  rst=off  init_reg=0  en=off  latency=bram_latency  dbl_ovrd=off  optimize=Area  use_rpm=off  block_type=spram
      settings: xl_area=[0, 0, 0, 0, 0, 0, 0]  block_version=9.1.01
  dout : Outport
  wires:
  Constant2/1 -> Single Port RAM/3
  din/1 -> Single Port RAM/2
  Counter/1 -> Single Port RAM/1, Relational/1
  Single Port RAM/1 -> dout/1
  Relational/1 -> Counter/1
  delay/1 -> AddSub/1
  AddSub/1 -> Relational/2
  Constant1/1 -> AddSub/2

== system casper_library/Delays/delay_complex ==
  In1 : Inport
  c_to_ri : casper_library/Misc/c_to_ri  n_bits=18  bin_pt=17
      settings: AttributesFormatString=18_17 r/i
  delay1 : Subsystem  BlockChoice=delay_bram
      link override delay_bram: DelayLen=delay  bram_latency=bram_latency
      link override delay_slr: DelayLen=delay
      settings: AttributesFormatString=%<BlockChoice>  TemplateBlock=casper_library/Delays/delay  MemberBlocks=delay_bram,delay_slr
  delay2 : Subsystem  BlockChoice=delay_bram
      link override delay_bram: DelayLen=delay  bram_latency=bram_latency
      link override delay_slr: DelayLen=delay
      settings: AttributesFormatString=%<BlockChoice>  TemplateBlock=casper_library/Delays/delay  MemberBlocks=delay_bram,delay_slr
  ri_to_c : casper_library/Misc/ri_to_c
  Out1 : Outport
  wires:
  c_to_ri/1 -> delay1/1(In1)
  delay1/1(Out1) -> ri_to_c/1
  c_to_ri/2 -> delay2/1(In1)
  delay2/1(Out1) -> ri_to_c/2
  In1/1 -> c_to_ri/1
  ri_to_c/1 -> Out1/1

== system casper_library/Delays/delay_slr ==
  In1 : Inport
  delay_slr : xbsIndex_r4/Delay  en=off  latency=DelayLen  dbl_ovrd=off  reg_retiming=off  block_type=delay
      settings: xl_area=[0, 0, 0, 0, 0, 0, 0]  block_version=9.1.01
  Out1 : Outport
  wires:
  delay_slr/1 -> Out1/1
  In1/1 -> delay_slr/1

== system casper_library/Delays/partial_delay_prog ==
  delay : Inport
  In1 : Inport  Port=2
  In2 : Inport  Port=3
  In3 : Inport  Port=4
  In4 : Inport  Port=5
  Delay{1..4} (4 alike) : xbsIndex_r4/Delay  en=off  latency=1  dbl_ovrd=off  reg_retiming=off  block_type=delay
      settings: xl_area=[0, 0, 0, 0, 0, 0, 0]  block_version=9.1.01
  Mux{1..4} (4 alike) : xbsIndex_r4/Mux  inputs=4  en=off  latency=2  precision=Full  arith_type="Signed  (2's comp)"  n_bits=8  bin_pt=2  quantization=Truncate  overflow=Wrap  dbl_ovrd=off  block_type=mux
      settings: xl_area=[0, 0, 0, 0, 0, 0, 0]  block_version=9.1.01
  Out1 : Outport
  Out2 : Outport  Port=2
  Out3 : Outport  Port=3
  Out4 : Outport  Port=4
  wires:
  In1/1 -> Delay1/1, Mux2/5, Mux3/4, Mux4/3
  Mux1/1 -> Out1/1
  delay/1 -> Mux1/1, Mux2/1, Mux3/1, Mux4/1
  Delay1/1 -> Mux1/2
  In2/1 -> Delay2/1, Mux3/5, Mux4/4
  Mux2/1 -> Out2/1
  Delay2/1 -> Mux2/2, Mux1/3
  In3/1 -> Delay3/1, Mux4/5
  Mux3/1 -> Out3/1
  Delay3/1 -> Mux3/2, Mux1/4, Mux2/3
  In4/1 -> Delay4/1
  Mux4/1 -> Out4/1
  Delay4/1 -> Mux4/2, Mux1/5, Mux2/4, Mux3/3

== system casper_library/Delays/sync_delay ==
  In : Inport
  Constant : xbsIndex_r4/Constant  arith_type=Unsigned  const=1  n_bits=BitWidth  bin_pt=0  explicit_period=on  period=1  equ=P=C  opselect=C  inp2=PCIN>>17  opr=+  inp1=P  carry=CIN  dbl_ovrd=off  block_type=constant
      settings: block_version=9.1.01
  Constant1 : xbsIndex_r4/Constant  arith_type=Unsigned  const=0  n_bits=BitWidth  bin_pt=0  explicit_period=on  period=1  equ=P=C  opselect=C  inp2=PCIN>>17  opr=+  inp1=P  carry=CIN  dbl_ovrd=off  block_type=constant
      settings: block_version=9.1.01
  Constant2 : xbsIndex_r4/Constant  arith_type=Unsigned  const=DelayLen  n_bits=BitWidth  bin_pt=0  explicit_period=on  period=1  equ=P=C  opselect=C  inp2=PCIN>>17  opr=+  inp1=P  carry=CIN  dbl_ovrd=off  block_type=constant
      settings: block_version=9.1.01
  Constant3 : xbsIndex_r4/Constant  arith_type=Unsigned  const=UseCounter  n_bits=1  bin_pt=0  explicit_period=on  period=1  equ=P=C  opselect=C  inp2=PCIN>>17  opr=+  inp1=P  carry=CIN  dbl_ovrd=off  block_type=constant
      settings: block_version=9.1.01
  Counter : xbsIndex_r4/Counter  cnt_type=Free Running  cnt_to=Inf  operation=Down  start_count=0  cnt_by_val=1  arith_type=Unsigned  n_bits=BitWidth  bin_pt=0  load_pin=on  rst=off  en=on  explicit_period=on  period=1  dbl_ovrd=off  use_behavioral_HDL=off  use_rpm=on  block_type=counter
      settings: xl_area=[0, 0, 0, 0, 0, 0, 0]  block_version=9.1.01
  Logical : xbsIndex_r4/Logical  logical_function=OR  inputs=2  en=off  latency=0  precision=Full  arith_type=Unsigned  n_bits=8  bin_pt=2  align_bp=on  dbl_ovrd=off  block_type=logical
      settings: xl_area=[0, 0, 0, 0, 0, 0, 0]  block_version=9.1.01
  Mux : xbsIndex_r4/Mux  inputs=2  en=off  latency=0  precision=Full  arith_type="Signed  (2's comp)"  n_bits=8  bin_pt=2  quantization=Truncate  overflow=Wrap  dbl_ovrd=off  block_type=mux
      settings: xl_area=[0, 0, 0, 0, 0, 0, 0]  block_version=9.1.01
  Relational : xbsIndex_r4/Relational  mode=a=b  en=off  latency=0  dbl_ovrd=off  block_type=relational
      settings: xl_area=[0, 0, 0, 0, 0, 0, 0]  block_version=9.1.01
  Relational1 : xbsIndex_r4/Relational  mode=a!=b  en=off  latency=0  dbl_ovrd=off  block_type=relational
      settings: xl_area=[0, 0, 0, 0, 0, 0, 0]  block_version=9.1.01
  warn period Logical0 : xbsReplacements_r4/Warning  SystemSampleTime=-1  period=1
  warn period Relational10 : xbsReplacements_r4/Warning  SystemSampleTime=-1  period=1
  Out : Outport
  wires:
  Mux/1 -> Out/1
  Constant3/1 -> Mux/1
  Relational/1 -> Mux/3
  Relational1/1 -> Logical/2
  Logical/1 -> Counter/3
  In/1 -> Mux/2, Logical/1, Counter/1
  Constant2/1 -> Counter/2
  Constant/1 -> Relational/1
  Constant1/1 -> Relational1/2
  Counter/1 -> Relational/2, Relational1/1

== system casper_library/Delays/sync_delay_en ==
  In : Inport
  en : Inport  Port=2
  Constant : xbsIndex_r4/Constant  arith_type=Unsigned  const=1  n_bits=BitWidth  bin_pt=0  explicit_period=on  period=1  equ=P=C  opselect=C  inp2=PCIN>>17  opr=+  inp1=P  carry=CIN  dbl_ovrd=off  block_type=constant
      settings: block_version=9.1.01
  Constant1 : xbsIndex_r4/Constant  arith_type=Unsigned  const=0  n_bits=BitWidth  bin_pt=0  explicit_period=on  period=1  equ=P=C  opselect=C  inp2=PCIN>>17  opr=+  inp1=P  carry=CIN  dbl_ovrd=off  block_type=constant
      settings: block_version=9.1.01
  Constant2 : xbsIndex_r4/Constant  arith_type=Unsigned  const=DelayLen  n_bits=BitWidth  bin_pt=0  explicit_period=on  period=1  equ=P=C  opselect=C  inp2=PCIN>>17  opr=+  inp1=P  carry=CIN  dbl_ovrd=off  block_type=constant
      settings: block_version=9.1.01
  Constant3 : xbsIndex_r4/Constant  arith_type=Unsigned  const=UseCounter  n_bits=1  bin_pt=0  explicit_period=on  period=1  equ=P=C  opselect=C  inp2=PCIN>>17  opr=+  inp1=P  carry=CIN  dbl_ovrd=off  block_type=constant
      settings: block_version=9.1.01
  Counter : xbsIndex_r4/Counter  cnt_type=Free Running  cnt_to=Inf  operation=Down  start_count=0  cnt_by_val=1  arith_type=Unsigned  n_bits=BitWidth  bin_pt=0  load_pin=on  rst=off  en=on  explicit_period=on  period=1  dbl_ovrd=off  use_behavioral_HDL=off  use_rpm=on  block_type=counter
      settings: xl_area=[0, 0, 0, 0, 0, 0, 0]  block_version=9.1.01
  Logical : xbsIndex_r4/Logical  logical_function=OR  inputs=2  en=off  latency=0  precision=Full  arith_type=Unsigned  n_bits=8  bin_pt=2  align_bp=on  dbl_ovrd=off  block_type=logical
      settings: xl_area=[0, 0, 0, 0, 0, 0, 0]  block_version=9.1.01
  Logical1 : xbsIndex_r4/Logical  logical_function=AND  inputs=2  en=off  latency=0  precision=Full  arith_type=Unsigned  n_bits=8  bin_pt=2  align_bp=on  dbl_ovrd=off  block_type=logical
      settings: xl_area=[0, 0, 0, 0, 0, 0, 0]  block_version=9.1.01
  Mux : xbsIndex_r4/Mux  inputs=2  en=off  latency=0  precision=Full  arith_type="Signed  (2's comp)"  n_bits=8  bin_pt=2  quantization=Truncate  overflow=Wrap  dbl_ovrd=off  block_type=mux
      settings: xl_area=[0, 0, 0, 0, 0, 0, 0]  block_version=9.1.01
  Relational : xbsIndex_r4/Relational  mode=a=b  en=off  latency=0  dbl_ovrd=off  block_type=relational
      settings: xl_area=[0, 0, 0, 0, 0, 0, 0]  block_version=9.1.01
  Relational1 : xbsIndex_r4/Relational  mode=a!=b  en=off  latency=0  dbl_ovrd=off  block_type=relational
      settings: xl_area=[0, 0, 0, 0, 0, 0, 0]  block_version=9.1.01
  warn period Logical0 : xbsReplacements_r4/Warning  SystemSampleTime=-1  period=1
  warn period Logical10 : xbsReplacements_r4/Warning  SystemSampleTime=-1  period=1
  warn period Relational10 : xbsReplacements_r4/Warning  SystemSampleTime=-1  period=1
  Out : Outport
  wires:
  Counter/1 -> Relational1/1, Relational/2
  Constant1/1 -> Relational1/2
  Constant/1 -> Relational/1
  Constant2/1 -> Counter/2
  In/1 -> Counter/1, Logical/1, Mux/2
  Relational1/1 -> Logical/2
  Relational/1 -> Mux/3
  Constant3/1 -> Mux/1
  Mux/1 -> Out/1
  Logical/1 -> Logical1/1
  Logical1/1 -> Counter/3
  en/1 -> Logical1/2

== system casper_library/Delays/sync_delay_prog ==
  sync : Inport
  delay : Inport  Port=2
  Constant : xbsIndex_r4/Constant  arith_type=Unsigned  const=1  n_bits=MaxDelay  bin_pt=0  explicit_period=on  period=1  equ=P=C  opselect=C  inp2=PCIN>>17  opr=+  inp1=P  carry=CIN  dbl_ovrd=off  block_type=constant
      settings: block_version=9.1.01
  Constant1 : xbsIndex_r4/Constant  arith_type=Unsigned  const=0  n_bits=MaxDelay  bin_pt=0  explicit_period=on  period=1  equ=P=C  opselect=C  inp2=PCIN>>17  opr=+  inp1=P  carry=CIN  dbl_ovrd=off  block_type=constant
      settings: block_version=9.1.01
  Counter : xbsIndex_r4/Counter  cnt_type=Free Running  cnt_to=Inf  operation=Down  start_count=0  cnt_by_val=1  arith_type=Unsigned  n_bits=MaxDelay  bin_pt=0  load_pin=on  rst=off  en=on  explicit_period=on  period=1  dbl_ovrd=off  use_behavioral_HDL=off  use_rpm=on  block_type=counter
      settings: xl_area=[0, 0, 0, 0, 0, 0, 0]  block_version=9.1.01
  Logical : xbsIndex_r4/Logical  logical_function=OR  inputs=2  en=off  latency=0  precision=Full  arith_type=Unsigned  n_bits=8  bin_pt=2  align_bp=on  dbl_ovrd=off  block_type=logical
      settings: xl_area=[0, 0, 0, 0, 0, 0, 0]  block_version=9.1.01
  Relational : xbsIndex_r4/Relational  mode=a=b  en=off  latency=0  dbl_ovrd=off  block_type=relational
      settings: xl_area=[0, 0, 0, 0, 0, 0, 0]  block_version=9.1.01
  Relational1 : xbsIndex_r4/Relational  mode=a!=b  en=off  latency=0  dbl_ovrd=off  block_type=relational
      settings: xl_area=[0, 0, 0, 0, 0, 0, 0]  block_version=9.1.01
  sync_out : Outport
  wires:
  Counter/1 -> Relational1/1, Relational/2
  Constant1/1 -> Relational1/2
  Constant/1 -> Relational/1
  delay/1 -> Counter/2
  sync/1 -> Counter/1, Logical/1
  Logical/1 -> Counter/3
  Relational1/1 -> Logical/2
  Relational/1 -> sync_out/1

== system casper_library/Downconverter/dds ==
  lo_const0 : casper_library/Downconverter/lo_const  SystemSampleTime=-1  n_bits=8  phase=0
  lo_const1 : casper_library/Downconverter/lo_const  SystemSampleTime=-1  n_bits=8  phase=1.5708
  lo_const2 : casper_library/Downconverter/lo_const  SystemSampleTime=-1  n_bits=8  phase=3.1416
  lo_const3 : casper_library/Downconverter/lo_const  SystemSampleTime=-1  n_bits=8  phase=4.7124
  sin0 : Outport
  cos0 : Outport  Port=2
  sin1 : Outport  Port=3
  cos1 : Outport  Port=4
  sin2 : Outport  Port=5
  cos2 : Outport  Port=6
  sin3 : Outport  Port=7
  cos3 : Outport  Port=8
  wires:
  lo_const0/1 -> sin0/1
  lo_const0/2 -> cos0/1
  lo_const1/1 -> sin1/1
  lo_const1/2 -> cos1/1
  lo_const2/1 -> sin2/1
  lo_const2/2 -> cos2/1
  lo_const3/1 -> sin3/1
  lo_const3/2 -> cos3/1

== system casper_library/Downconverter/dec_fir ==
  sync_in : Inport
  real1 : Inport  Port=2
  imag1 : Inport  Port=3
  real2 : Inport  Port=4
  imag2 : Inport  Port=5
  convert1 : xbsIndex_r4/Convert  arith_type="Signed  (2's comp)"  n_bits=4  bin_pt=3  quantization=Truncate  overflow=Saturate  latency=3  dbl_ovrd=off  pipeline=on  block_type=convert
      settings: xl_area=[0, 0, 0, 0, 0, 0, 0]
  convert2 : xbsIndex_r4/Convert  arith_type="Signed  (2's comp)"  n_bits=4  bin_pt=3  quantization=Truncate  overflow=Saturate  latency=3  dbl_ovrd=off  pipeline=on  block_type=convert
      settings: xl_area=[0, 0, 0, 0, 0, 0, 0]
  delay : xbsIndex_r4/Delay  en=off  latency=49  dbl_ovrd=off  reg_retiming=off  block_type=delay
      settings: xl_area=[0, 0, 0, 0, 0, 0, 0]  block_version=9.1.01
  fir_col1 : Subsystem  AncestorBlock=casper_library/Downconverter/fir_col  mask(fir_col){n_inputs=2, coeff=[5 4], add_latency=2, mult_latency=45}
      mask prompts: n_inputs "Inputs"; coeff "Coefficients"; add_latency "Add latency"; mult_latency "Mult Latency"
      mask init:
      | fir_col_init(gcb, ...
      |     'n_inputs', n_inputs,...
      |     'coeff', coeff, ...
      |     'mult_latency', mult_latency, ...
      |     'add_latency', add_latency);
  imag_sum : Subsystem  AncestorBlock=casper_library/Misc/adder_tree  mask(adder_tree){n_inputs=1, latency=3}
      mask prompts: n_inputs "Number of Inputs"; latency "Add Latency"
      mask help: Sums all inputs using a tree of adds and delays.
      mask init:
      | adder_tree_init(gcb, ...
      |     'n_inputs', n_inputs, ...
      |     'latency', latency);
      settings: AttributesFormatString=latency 0
      mask Help: eval('xlWeb([getenv(''MLIB_ROOT''), ''\doc\html\sp_adder_tree\sp_adder_tree.html''])')
  real_sum : Subsystem  AncestorBlock=casper_library/Misc/adder_tree  mask(adder_tree){n_inputs=1, latency=3}
      mask prompts: n_inputs "Number of Inputs"; latency "Add Latency"
      mask help: Sums all inputs using a tree of adds and delays.
      mask init:
      | adder_tree_init(gcb, ...
      |     'n_inputs', n_inputs, ...
      |     'latency', latency);
      settings: AttributesFormatString=latency 0
      mask Help: eval('xlWeb([getenv(''MLIB_ROOT''), ''\doc\html\sp_adder_tree\sp_adder_tree.html''])')
  ri_to_c : Subsystem
  shift1 : xbsIndex_r4/Shift  shift_dir=Left  shift_bits=1  en=off  latency=0  precision=Full  arith_type="Signed  (2's comp)"  n_bits=8  bin_pt=2  quantization=Truncate  overflow=Wrap  dbl_ovrd=off  block_type=shift
      settings: xl_area=[0, 0, 0, 0, 0, 0, 0]  block_version=9.1.01
  shift2 : xbsIndex_r4/Shift  shift_dir=Left  shift_bits=1  en=off  latency=0  precision=Full  arith_type="Signed  (2's comp)"  n_bits=8  bin_pt=2  quantization=Truncate  overflow=Wrap  dbl_ovrd=off  block_type=shift
      settings: xl_area=[0, 0, 0, 0, 0, 0, 0]  block_version=9.1.01
  sync_out : Outport
  dout : Outport  Port=2
  wires:
  real_sum/1(sync_out) -> sync_out/1
  delay/1 -> imag_sum/1(sync), real_sum/1(sync)
  sync_in/1 -> delay/1
  ri_to_c/1(c) -> dout/1
  convert2/1 -> ri_to_c/2(im)
  convert1/1 -> ri_to_c/1(re)
  shift2/1 -> convert2/1
  shift1/1 -> convert1/1
  imag_sum/2(dout) -> shift2/1
  real_sum/2(dout) -> shift1/1
  fir_col1/6(imag_sum) -> imag_sum/2(din1)
  fir_col1/5(real_sum) -> real_sum/2(din1)
  imag2/1 -> fir_col1/4(imag2)
  real2/1 -> fir_col1/3(real2)
  imag1/1 -> fir_col1/2(imag1)
  real1/1 -> fir_col1/1(real1)
